simulink model "controlNN"  (R2020b)
settings: Solver=VariableStepAuto  StartTime=0.0  StopTime=50  RelTol=1e-3
undefined symbols (not defined in the file): DiscIntNeverNeededParam, FF_L, FF_R, initial_uspeed, Kih, Kir
libraries: neural x116, simulink x4, simulink_extras x3, dspsrcs4 x1, pid_lib x1
(part 2 of 5)

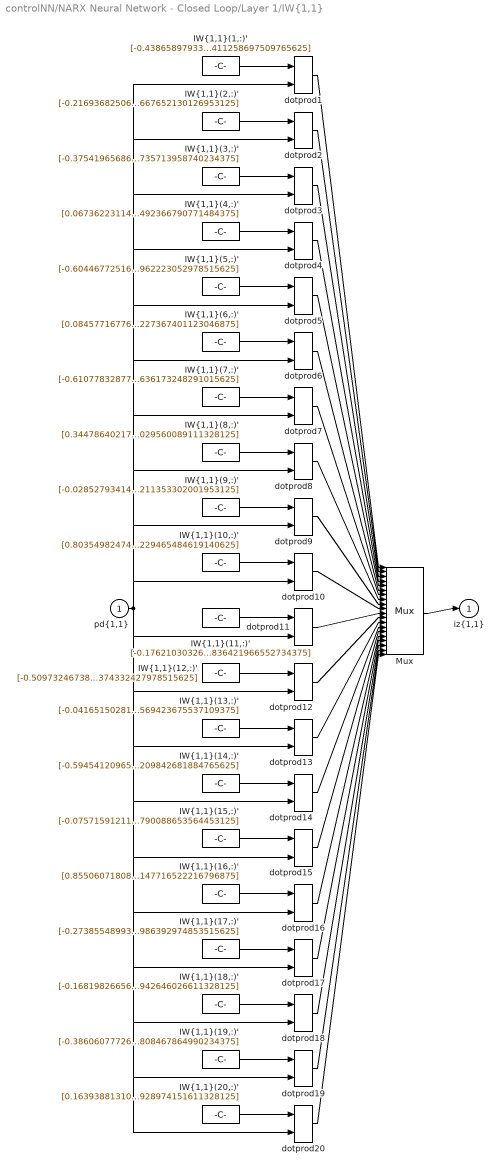
== system controlNN/NARX Neural Network - Closed Loop/Layer 1/IW{1,1} ==
  "pd{1,1}" : Inport  PortDimensions=4  SampleTime=0.1
      mask Display: e = 0.06;c1 = [120 230 180]/255;c2 = ([120 230 180]+0)/(256+128);c3 = ([120 230 180]+128)/(256+128);patch([0 1 1 0],[0 0 1 1],c1);patch([0 1 1 1-e 1-e 0+e],[0 0 1 1-e 0+e 0+e],c2);patch([0 0 1 1-e 0+e 0+e],[0 1 1 1-e 1-e 0+e],c3);plot([0 1 1 0 0],[0 0 1 1 0]);
  "IW{1,1}(1,:)'" : Constant  Value=[-0.4386589793372710488483789958991110324859619140625;-0.018740802820601483447138235760576208122074604034423828125;0.417644650165202413472087528134579770267009735107421875;-0.11303759033649586618341942312326864339411258697509765625]
      mask Display: e = 0.06;c1 = [120 150 230]/255;c2 = ([120 150 230]+0)/383;c3 = ([120 150 230]+128)/383;patch([0 1 1 0],[0 0 1 1],c1);patch([0 1 1 1-e 1-e 0+e],[0 0 1 1-e 0+e 0+e],c2);patch([0 0 1 1-e 0+e 0+e],[0 1 1 1-e 1-e 0+e],c3);plot([0 1 1 0 0],[0 0 1 1 0]);disp('Weights');
  "IW{1,1}(10,:)'" : Constant  Value=[0.8035498247491827950028664417914114892482757568359375;-0.852615893781887290714394112001173198223114013671875;0.029692839364198787832638259942541480995714664459228515625;0.131333870605793878727496348801651038229465484619140625]
      mask Display: e = 0.06;c1 = [120 150 230]/255;c2 = ([120 150 230]+0)/383;c3 = ([120 150 230]+128)/383;patch([0 1 1 0],[0 0 1 1],c1);patch([0 1 1 1-e 1-e 0+e],[0 0 1 1-e 0+e 0+e],c2);patch([0 0 1 1-e 0+e 0+e],[0 1 1 1-e 1-e 0+e],c3);plot([0 1 1 0 0],[0 0 1 1 0]);disp('Weights');
  "IW{1,1}(11,:)'" : Constant  Value=[-0.176210303269895229849595352789037860929965972900390625;0.3631567673090703163296666389214806258678436279296875;0.00443034452357003206979246812124983989633619785308837890625;-0.279013486365463359017979882992221973836421966552734375]
      mask Display: e = 0.06;c1 = [120 150 230]/255;c2 = ([120 150 230]+0)/383;c3 = ([120 150 230]+128)/383;patch([0 1 1 0],[0 0 1 1],c1);patch([0 1 1 1-e 1-e 0+e],[0 0 1 1-e 0+e 0+e],c2);patch([0 0 1 1-e 0+e 0+e],[0 1 1 1-e 1-e 0+e],c3);plot([0 1 1 0 0],[0 0 1 1 0]);disp('Weights');
  "IW{1,1}(12,:)'" : Constant  Value=[-0.50973246738134780908779930541641078889369964599609375;0.1274233060214269019905231061784434132277965545654296875;-0.03424515071449614478371614723073435015976428985595703125;-0.0299313497305035459972177847021157504059374332427978515625]
      mask Display: e = 0.06;c1 = [120 150 230]/255;c2 = ([120 150 230]+0)/383;c3 = ([120 150 230]+128)/383;patch([0 1 1 0],[0 0 1 1],c1);patch([0 1 1 1-e 1-e 0+e],[0 0 1 1-e 0+e 0+e],c2);patch([0 0 1 1-e 0+e 0+e],[0 1 1 1-e 1-e 0+e],c3);plot([0 1 1 0 0],[0 0 1 1 0]);disp('Weights');
  "IW{1,1}(13,:)'" : Constant  Value=[-0.041651502817647630128039537567019579000771045684814453125;-0.10168864752925420302798187321968725882470607757568359375;-0.14637329203365190277708052235539071261882781982421875;-0.3056214640627208378731438642716966569423675537109375]
      mask Display: e = 0.06;c1 = [120 150 230]/255;c2 = ([120 150 230]+0)/383;c3 = ([120 150 230]+128)/383;patch([0 1 1 0],[0 0 1 1],c1);patch([0 1 1 1-e 1-e 0+e],[0 0 1 1-e 0+e 0+e],c2);patch([0 0 1 1-e 0+e 0+e],[0 1 1 1-e 1-e 0+e],c3);plot([0 1 1 0 0],[0 0 1 1 0]);disp('Weights');
  "IW{1,1}(14,:)'" : Constant  Value=[-0.59454120965693724176759360489086247980594635009765625;0.187929342664180765165582442932645790278911590576171875;0.174064349978933885498832978555583395063877105712890625;-0.53969192686360278887747199405566789209842681884765625]
      mask Display: e = 0.06;c1 = [120 150 230]/255;c2 = ([120 150 230]+0)/383;c3 = ([120 150 230]+128)/383;patch([0 1 1 0],[0 0 1 1],c1);patch([0 1 1 1-e 1-e 0+e],[0 0 1 1-e 0+e 0+e],c2);patch([0 0 1 1-e 0+e 0+e],[0 1 1 1-e 1-e 0+e],c3);plot([0 1 1 0 0],[0 0 1 1 0]);disp('Weights');
  "IW{1,1}(15,:)'" : Constant  Value=[-0.07571591211695156975469700455505517311394214630126953125;0.407648907576858565704469583579339087009429931640625;0.017529421576475530397676294569464516825973987579345703125;-0.2305489952766562045116671697542187757790088653564453125]
      mask Display: e = 0.06;c1 = [120 150 230]/255;c2 = ([120 150 230]+0)/383;c3 = ([120 150 230]+128)/383;patch([0 1 1 0],[0 0 1 1],c1);patch([0 1 1 1-e 1-e 0+e],[0 0 1 1-e 0+e 0+e],c2);patch([0 0 1 1-e 0+e 0+e],[0 1 1 1-e 1-e 0+e],c3);plot([0 1 1 0 0],[0 0 1 1 0]);disp('Weights');
  "IW{1,1}(16,:)'" : Constant  Value=[0.8550607180854485900312056401162408292293548583984375;-0.76669221688588040652945210240432061254978179931640625;-0.330474331205291294022430292898206971585750579833984375;1.144481090073003581863986255484633147716522216796875]
      mask Display: e = 0.06;c1 = [120 150 230]/255;c2 = ([120 150 230]+0)/383;c3 = ([120 150 230]+128)/383;patch([0 1 1 0],[0 0 1 1],c1);patch([0 1 1 1-e 1-e 0+e],[0 0 1 1-e 0+e 0+e],c2);patch([0 0 1 1-e 0+e 0+e],[0 1 1 1-e 1-e 0+e],c3);plot([0 1 1 0 0],[0 0 1 1 0]);disp('Weights');
  "IW{1,1}(17,:)'" : Constant  Value=[-0.273855489939183183167870083707384765148162841796875;0.73849739533944214198157851569703780114650726318359375;-0.161805029543822309623379851473146118223667144775390625;-0.376344550552319800917899783598841167986392974853515625]
      mask Display: e = 0.06;c1 = [120 150 230]/255;c2 = ([120 150 230]+0)/383;c3 = ([120 150 230]+128)/383;patch([0 1 1 0],[0 0 1 1],c1);patch([0 1 1 1-e 1-e 0+e],[0 0 1 1-e 0+e 0+e],c2);patch([0 0 1 1-e 0+e 0+e],[0 1 1 1-e 1-e 0+e],c3);plot([0 1 1 0 0],[0 0 1 1 0]);disp('Weights');
  "IW{1,1}(18,:)'" : Constant  Value=[-0.1681982665624602024667666455570724792778491973876953125;0.1950333915332860268421200089505873620510101318359375;0.325788197182866390289035507521475665271282196044921875;0.38078155832405713443478134649922139942646026611328125]
      mask Display: e = 0.06;c1 = [120 150 230]/255;c2 = ([120 150 230]+0)/383;c3 = ([120 150 230]+128)/383;patch([0 1 1 0],[0 0 1 1],c1);patch([0 1 1 1-e 1-e 0+e],[0 0 1 1-e 0+e 0+e],c2);patch([0 0 1 1-e 0+e 0+e],[0 1 1 1-e 1-e 0+e],c3);plot([0 1 1 0 0],[0 0 1 1 0]);disp('Weights');
  "IW{1,1}(19,:)'" : Constant  Value=[-0.3860607772679796045878219956648536026477813720703125;0.005620361738486860138375167394997333758510649204254150390625;-0.2093565241992116632285814148417557589709758758544921875;0.203667618207004019748040946069522760808467864990234375]
      mask Display: e = 0.06;c1 = [120 150 230]/255;c2 = ([120 150 230]+0)/383;c3 = ([120 150 230]+128)/383;patch([0 1 1 0],[0 0 1 1],c1);patch([0 1 1 1-e 1-e 0+e],[0 0 1 1-e 0+e 0+e],c2);patch([0 0 1 1-e 0+e 0+e],[0 1 1 1-e 1-e 0+e],c3);plot([0 1 1 0 0],[0 0 1 1 0]);disp('Weights');
  "IW{1,1}(2,:)'" : Constant  Value=[-0.2169368250631043271159370533496257849037647247314453125;-0.10077498959220541896453227082020021043717861175537109375;0.2530416473236523078327309121959842741489410400390625;0.66912441916586662404853314001229591667652130126953125]
      mask Display: e = 0.06;c1 = [120 150 230]/255;c2 = ([120 150 230]+0)/383;c3 = ([120 150 230]+128)/383;patch([0 1 1 0],[0 0 1 1],c1);patch([0 1 1 1-e 1-e 0+e],[0 0 1 1-e 0+e 0+e],c2);patch([0 0 1 1-e 0+e 0+e],[0 1 1 1-e 1-e 0+e],c3);plot([0 1 1 0 0],[0 0 1 1 0]);disp('Weights');
  "IW{1,1}(20,:)'" : Constant  Value=[0.1639388131040236118440844848009874112904071807861328125;-0.11483736125112457837627033541139098815619945526123046875;-0.2099411749306478169874168315800488926470279693603515625;0.08683169221030291595742056642848183400928974151611328125]
      mask Display: e = 0.06;c1 = [120 150 230]/255;c2 = ([120 150 230]+0)/383;c3 = ([120 150 230]+128)/383;patch([0 1 1 0],[0 0 1 1],c1);patch([0 1 1 1-e 1-e 0+e],[0 0 1 1-e 0+e 0+e],c2);patch([0 0 1 1-e 0+e 0+e],[0 1 1 1-e 1-e 0+e],c3);plot([0 1 1 0 0],[0 0 1 1 0]);disp('Weights');
  "IW{1,1}(3,:)'" : Constant  Value=[-0.37541965686606160179650260033668018877506256103515625;-0.20153178909663049811484825113439001142978668212890625;-0.466435294275771183958312349204788915812969207763671875;0.33277599345324071489216066765948198735713958740234375]
      mask Display: e = 0.06;c1 = [120 150 230]/255;c2 = ([120 150 230]+0)/383;c3 = ([120 150 230]+128)/383;patch([0 1 1 0],[0 0 1 1],c1);patch([0 1 1 1-e 1-e 0+e],[0 0 1 1-e 0+e 0+e],c2);patch([0 0 1 1-e 0+e 0+e],[0 1 1 1-e 1-e 0+e],c3);plot([0 1 1 0 0],[0 0 1 1 0]);disp('Weights');
  "IW{1,1}(4,:)'" : Constant  Value=[0.0673622311467110268523583727073855698108673095703125;-0.486251970232177532782458229121402837336063385009765625;-0.06241567356591477822025382238280144520103931427001953125;0.402933162705098213418608565916656516492366790771484375]
      mask Display: e = 0.06;c1 = [120 150 230]/255;c2 = ([120 150 230]+0)/383;c3 = ([120 150 230]+128)/383;patch([0 1 1 0],[0 0 1 1],c1);patch([0 1 1 1-e 1-e 0+e],[0 0 1 1-e 0+e 0+e],c2);patch([0 0 1 1-e 0+e 0+e],[0 1 1 1-e 1-e 0+e],c3);plot([0 1 1 0 0],[0 0 1 1 0]);disp('Weights');
  "IW{1,1}(5,:)'" : Constant  Value=[-0.6044677251635601766821537239593453705310821533203125;0.59556534702274677162137095365324057638645172119140625;-0.2165999782456699274124645171468728221952915191650390625;-0.32745838498189228094048530692816711962223052978515625]
      mask Display: e = 0.06;c1 = [120 150 230]/255;c2 = ([120 150 230]+0)/383;c3 = ([120 150 230]+128)/383;patch([0 1 1 0],[0 0 1 1],c1);patch([0 1 1 1-e 1-e 0+e],[0 0 1 1-e 0+e 0+e],c2);patch([0 0 1 1-e 0+e 0+e],[0 1 1 1-e 1-e 0+e],c3);plot([0 1 1 0 0],[0 0 1 1 0]);disp('Weights');
  "IW{1,1}(6,:)'" : Constant  Value=[0.08457716776205737030380760188563726842403411865234375;0.164731897714957831180271341509069316089153289794921875;0.06115368927873300608499818054042407311499118804931640625;-0.162399602033176104765033187504741363227367401123046875]
      mask Display: e = 0.06;c1 = [120 150 230]/255;c2 = ([120 150 230]+0)/383;c3 = ([120 150 230]+128)/383;patch([0 1 1 0],[0 0 1 1],c1);patch([0 1 1 1-e 1-e 0+e],[0 0 1 1-e 0+e 0+e],c2);patch([0 0 1 1-e 0+e 0+e],[0 1 1 1-e 1-e 0+e],c3);plot([0 1 1 0 0],[0 0 1 1 0]);disp('Weights');
  "IW{1,1}(7,:)'" : Constant  Value=[-0.6107783287765347068898336146958172321319580078125;0.056990451234282736570069261006210581399500370025634765625;-0.164006181104764670042328589261160232126712799072265625;-0.0957481372975642897049652901841909624636173248291015625]
      mask Display: e = 0.06;c1 = [120 150 230]/255;c2 = ([120 150 230]+0)/383;c3 = ([120 150 230]+128)/383;patch([0 1 1 0],[0 0 1 1],c1);patch([0 1 1 1-e 1-e 0+e],[0 0 1 1-e 0+e 0+e],c2);patch([0 0 1 1-e 0+e 0+e],[0 1 1 1-e 1-e 0+e],c3);plot([0 1 1 0 0],[0 0 1 1 0]);disp('Weights');
  "IW{1,1}(8,:)'" : Constant  Value=[0.34478640217807143830697214070823974907398223876953125;-0.496796585967090920110678098353673703968524932861328125;-0.067509984111881971013957581817521713674068450927734375;0.3095067145511365414023430275847204029560089111328125]
      mask Display: e = 0.06;c1 = [120 150 230]/255;c2 = ([120 150 230]+0)/383;c3 = ([120 150 230]+128)/383;patch([0 1 1 0],[0 0 1 1],c1);patch([0 1 1 1-e 1-e 0+e],[0 0 1 1-e 0+e 0+e],c2);patch([0 0 1 1-e 0+e 0+e],[0 1 1 1-e 1-e 0+e],c3);plot([0 1 1 0 0],[0 0 1 1 0]);disp('Weights');
  "IW{1,1}(9,:)'" : Constant  Value=[-0.02852793414041586428364638550192466937005519866943359375;0.1993846370832842718190391906318836845457553863525390625;-0.1083183159449141730323873389352229423820972442626953125;-0.18780342166301100537140200685826130211353302001953125]
      mask Display: e = 0.06;c1 = [120 150 230]/255;c2 = ([120 150 230]+0)/383;c3 = ([120 150 230]+128)/383;patch([0 1 1 0],[0 0 1 1],c1);patch([0 1 1 1-e 1-e 0+e],[0 0 1 1-e 0+e 0+e],c2);patch([0 0 1 1-e 0+e 0+e],[0 1 1 1-e 1-e 0+e],c3);plot([0 1 1 0 0],[0 0 1 1 0]);disp('Weights');
  Mux : Mux  Inputs=20
      mask Display: e = 0.06;c1 = [120 150 230]/255;c2 = ([120 150 230]+0)/383;c3 = ([120 150 230]+128)/383;patch([0 1 1 0],[0 0 1 1],c1);patch([0 1 1 1-e 1-e 0+e],[0 0 1 1-e 0+e 0+e],c2);patch([0 0 1 1-e 0+e 0+e],[0 1 1 1-e 1-e 0+e],c3);plot([0 1 1 0 0],[0 0 1 1 0]);disp('Mux');
  dotprod{1..20} (20 alike) : neural/Weight Functions/dotprod
  "iz{1,1}" : Outport
      mask Display: e = 0.06;c1 = [120 230 180]/255;c2 = ([120 230 180]+0)/(256+128);c3 = ([120 230 180]+128)/(256+128);patch([0 1 1 0],[0 0 1 1],c1);patch([0 1 1 1-e 1-e 0+e],[0 0 1 1-e 0+e 0+e],c2);patch([0 0 1 1-e 0+e 0+e],[0 1 1 1-e 1-e 0+e],c3);plot([0 1 1 0 0],[0 0 1 1 0]);
  wires:
  "IW{1,1}(1,:)'"/1 -> dotprod1/1
  "pd{1,1}"/1 -> dotprod1/2, dotprod2/2, dotprod3/2, dotprod4/2, dotprod5/2, dotprod6/2, dotprod7/2, dotprod8/2, dotprod9/2, dotprod10/2, dotprod11/2, dotprod12/2, dotprod13/2, dotprod14/2, dotprod15/2, dotprod16/2, dotprod17/2, dotprod18/2, dotprod19/2, dotprod20/2
  dotprod1/1 -> Mux/1
  "IW{1,1}(2,:)'"/1 -> dotprod2/1
  dotprod2/1 -> Mux/2
  "IW{1,1}(3,:)'"/1 -> dotprod3/1
  dotprod3/1 -> Mux/3
  "IW{1,1}(4,:)'"/1 -> dotprod4/1
  dotprod4/1 -> Mux/4
  "IW{1,1}(5,:)'"/1 -> dotprod5/1
  dotprod5/1 -> Mux/5
  "IW{1,1}(6,:)'"/1 -> dotprod6/1
  dotprod6/1 -> Mux/6
  "IW{1,1}(7,:)'"/1 -> dotprod7/1
  dotprod7/1 -> Mux/7
  "IW{1,1}(8,:)'"/1 -> dotprod8/1
  dotprod8/1 -> Mux/8
  "IW{1,1}(9,:)'"/1 -> dotprod9/1
  dotprod9/1 -> Mux/9
  "IW{1,1}(10,:)'"/1 -> dotprod10/1
  dotprod10/1 -> Mux/10
  "IW{1,1}(11,:)'"/1 -> dotprod11/1
  dotprod11/1 -> Mux/11
  "IW{1,1}(12,:)'"/1 -> dotprod12/1
  dotprod12/1 -> Mux/12
  "IW{1,1}(13,:)'"/1 -> dotprod13/1
  dotprod13/1 -> Mux/13
  "IW{1,1}(14,:)'"/1 -> dotprod14/1
  dotprod14/1 -> Mux/14
  "IW{1,1}(15,:)'"/1 -> dotprod15/1
  dotprod15/1 -> Mux/15
  "IW{1,1}(16,:)'"/1 -> dotprod16/1
  dotprod16/1 -> Mux/16
  "IW{1,1}(17,:)'"/1 -> dotprod17/1
  dotprod17/1 -> Mux/17
  "IW{1,1}(18,:)'"/1 -> dotprod18/1
  dotprod18/1 -> Mux/18
  "IW{1,1}(19,:)'"/1 -> dotprod19/1
  dotprod19/1 -> Mux/19
  "IW{1,1}(20,:)'"/1 -> dotprod20/1
  dotprod20/1 -> Mux/20
  Mux/1 -> "iz{1,1}"/1

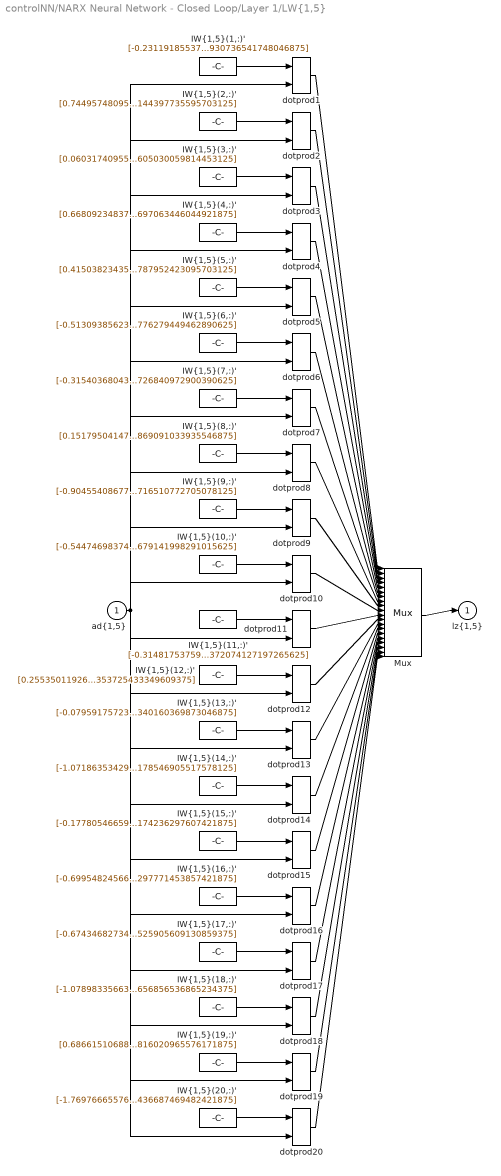
== system controlNN/NARX Neural Network - Closed Loop/Layer 1/LW{1,5} ==
  "ad{1,5}" : Inport  PortDimensions=9  SampleTime=0.1
      mask Display: e = 0.06;c1 = [120 230 180]/255;c2 = ([120 230 180]+0)/(256+128);c3 = ([120 230 180]+128)/(256+128);patch([0 1 1 0],[0 0 1 1],c1);patch([0 1 1 1-e 1-e 0+e],[0 0 1 1-e 0+e 0+e],c2);patch([0 0 1 1-e 0+e 0+e],[0 1 1 1-e 1-e 0+e],c3);plot([0 1 1 0 0],[0 0 1 1 0]);
  "IW{1,5}(1,:)'" : Constant  Value=[-0.2311918553757970062889626206015236675739288330078125;0.5221402736602007710331463385955430567264556884765625;0.0243916179590730301807166569005858036689460277557373046875;-0.217996142397916481403541411054902710020542144775390625;-0.1464474710870238005622212540401960723102092742919921875;0.5650549066626735505991518948576413094997406005859375;-0.023897965720476442574859987644231296144425868988037109375;0.11174950041300375780384257495825295336544513702392578125;0.73893306396338143127167086277040652930736541748046875]
      mask Display: e = 0.06;c1 = [120 150 230]/255;c2 = ([120 150 230]+0)/383;c3 = ([120 150 230]+128)/383;patch([0 1 1 0],[0 0 1 1],c1);patch([0 1 1 1-e 1-e 0+e],[0 0 1 1-e 0+e 0+e],c2);patch([0 0 1 1-e 0+e 0+e],[0 1 1 1-e 1-e 0+e],c3);plot([0 1 1 0 0],[0 0 1 1 0]);disp('weights');
  "IW{1,5}(10,:)'" : Constant  Value=[-0.544746983743852997150725059327669441699981689453125;-0.0208669004603495890359798892177423113025724887847900390625;-0.0390067613804046253722646042660926468670368194580078125;-0.284810235129842104218056419995264150202274322509765625;1.351958020913929914286200073547661304473876953125;0.162511610923024185648699813100392930209636688232421875;-0.22443140784391879538617331490968354046344757080078125;-0.06900460407357102143866001142669119872152805328369140625;0.8008568126875614812121284558088518679141998291015625]
      mask Display: e = 0.06;c1 = [120 150 230]/255;c2 = ([120 150 230]+0)/383;c3 = ([120 150 230]+128)/383;patch([0 1 1 0],[0 0 1 1],c1);patch([0 1 1 1-e 1-e 0+e],[0 0 1 1-e 0+e 0+e],c2);patch([0 0 1 1-e 0+e 0+e],[0 1 1 1-e 1-e 0+e],c3);plot([0 1 1 0 0],[0 0 1 1 0]);disp('weights');
  "IW{1,5}(11,:)'" : Constant  Value=[-0.3148175375952864119000196296838112175464630126953125;-0.0201252255988595106506178211702717817388474941253662109375;-0.041906260492351458946114206582933547906577587127685546875;0.3251339505202330837363433602149598300457000732421875;0.183494807709077945023778966060490347445011138916015625;-0.01587083282701005904069546659229672513902187347412109375;-0.270686784721715867352287432368029840290546417236328125;0.0331311256809694032465785085150855593383312225341796875;0.1110384185024998748847480101176188327372074127197265625]
      mask Display: e = 0.06;c1 = [120 150 230]/255;c2 = ([120 150 230]+0)/383;c3 = ([120 150 230]+128)/383;patch([0 1 1 0],[0 0 1 1],c1);patch([0 1 1 1-e 1-e 0+e],[0 0 1 1-e 0+e 0+e],c2);patch([0 0 1 1-e 0+e 0+e],[0 1 1 1-e 1-e 0+e],c3);plot([0 1 1 0 0],[0 0 1 1 0]);disp('weights');
  "IW{1,5}(12,:)'" : Constant  Value=[0.25535011926189488118410508832312189042568206787109375;-0.06781103850008314559705269175537978298962116241455078125;-0.1765333104449736401075909952851361595094203948974609375;-0.07995557032786904105847725077182985842227935791015625;-0.56790209529041202340948757409933023154735565185546875;0.12368783117214422750951285934206680394709110260009765625;-0.050807955374315115493200067930956720374524593353271484375;-0.1708000662816792358800199735924252308905124664306640625;-0.3310316189289499444470266098505817353725433349609375]
      mask Display: e = 0.06;c1 = [120 150 230]/255;c2 = ([120 150 230]+0)/383;c3 = ([120 150 230]+128)/383;patch([0 1 1 0],[0 0 1 1],c1);patch([0 1 1 1-e 1-e 0+e],[0 0 1 1-e 0+e 0+e],c2);patch([0 0 1 1-e 0+e 0+e],[0 1 1 1-e 1-e 0+e],c3);plot([0 1 1 0 0],[0 0 1 1 0]);disp('weights');
  "IW{1,5}(13,:)'" : Constant  Value=[-0.079591757232955473444491190093685872852802276611328125;0.26871266099311064134980142625863663852214813232421875;0.19483515376642579486343720418517477810382843017578125;0.2158877741672318439913880183667060919106006622314453125;-0.7479795700745845987711390989716164767742156982421875;0.64235516354538024774711857389775104820728302001953125;-0.301808244484936871732116969724302180111408233642578125;0.409133320230898822611464993315166793763637542724609375;-0.01345306195830124444678954631626766058616340160369873046875]
      mask Display: e = 0.06;c1 = [120 150 230]/255;c2 = ([120 150 230]+0)/383;c3 = ([120 150 230]+128)/383;patch([0 1 1 0],[0 0 1 1],c1);patch([0 1 1 1-e 1-e 0+e],[0 0 1 1-e 0+e 0+e],c2);patch([0 0 1 1-e 0+e 0+e],[0 1 1 1-e 1-e 0+e],c3);plot([0 1 1 0 0],[0 0 1 1 0]);disp('weights');
  "IW{1,5}(14,:)'" : Constant  Value=[-1.071863534293599595770274390815757215023040771484375;0.1989523045064365280865104068652726709842681884765625;0.220235805372647586164447375267627649009227752685546875;-0.41885820333493539724400989143759943544864654541015625;0.2410461404675325047808343015276477672159671783447265625;-0.0800863220582195278751669320627115666866302490234375;0.28295401326276181652730201676604337990283966064453125;0.72681780994764988435008490341715514659881591796875;-0.3208844679775921804321114905178546905517578125]
      mask Display: e = 0.06;c1 = [120 150 230]/255;c2 = ([120 150 230]+0)/383;c3 = ([120 150 230]+128)/383;patch([0 1 1 0],[0 0 1 1],c1);patch([0 1 1 1-e 1-e 0+e],[0 0 1 1-e 0+e 0+e],c2);patch([0 0 1 1-e 0+e 0+e],[0 1 1 1-e 1-e 0+e],c3);plot([0 1 1 0 0],[0 0 1 1 0]);disp('weights');
  "IW{1,5}(15,:)'" : Constant  Value=[-0.17780546659272411513796896542771719396114349365234375;-0.09782683516892017039356943541861255653202533721923828125;0.146761535994159475482234711307683028280735015869140625;0.08471415768842437132857270398744731210172176361083984375;0.54963220471845442016700644671800546348094940185546875;-0.0534051530097601478974667088550631888210773468017578125;0.07172658702519178752776696228465880267322063446044921875;-0.0810404904925203783960796499741263687610626220703125;-0.1615679641183165038409441649491782300174236297607421875]
      mask Display: e = 0.06;c1 = [120 150 230]/255;c2 = ([120 150 230]+0)/383;c3 = ([120 150 230]+128)/383;patch([0 1 1 0],[0 0 1 1],c1);patch([0 1 1 1-e 1-e 0+e],[0 0 1 1-e 0+e 0+e],c2);patch([0 0 1 1-e 0+e 0+e],[0 1 1 1-e 1-e 0+e],c3);plot([0 1 1 0 0],[0 0 1 1 0]);disp('weights');
  "IW{1,5}(16,:)'" : Constant  Value=[-0.6995482456630373047090643012779764831066131591796875;-0.52576189513835480671133382202242501080036163330078125;0.1860761240495697188546131428665830753743648529052734375;0.56796598824997868160124880887451581656932830810546875;0.91231789653880834833898916258476674556732177734375;0.171360138456032817799723488860763609409332275390625;-1.2741680689427834494154012645594775676727294921875;0.333742099312757556361930255661718547344207763671875;-0.0291920767385230144064234281131575698964297771453857421875]
      mask Display: e = 0.06;c1 = [120 150 230]/255;c2 = ([120 150 230]+0)/383;c3 = ([120 150 230]+128)/383;patch([0 1 1 0],[0 0 1 1],c1);patch([0 1 1 1-e 1-e 0+e],[0 0 1 1-e 0+e 0+e],c2);patch([0 0 1 1-e 0+e 0+e],[0 1 1 1-e 1-e 0+e],c3);plot([0 1 1 0 0],[0 0 1 1 0]);disp('weights');
  "IW{1,5}(17,:)'" : Constant  Value=[-0.67434682734431816708564610962639562785625457763671875;0.178838922670269628856232202451792545616626739501953125;-0.022826342936018338691805951157220988534390926361083984375;-0.2204262955518062894189057487892569042742252349853515625;0.785536261603020147248344073886983096599578857421875;-0.1615962577050045201332295619067735970020294189453125;-0.0093114199088808434490172061259727342985570430755615234375;-0.280812232310453990802301404983154498040676116943359375;-0.95914663710902414717196506899199448525905609130859375]
      mask Display: e = 0.06;c1 = [120 150 230]/255;c2 = ([120 150 230]+0)/383;c3 = ([120 150 230]+128)/383;patch([0 1 1 0],[0 0 1 1],c1);patch([0 1 1 1-e 1-e 0+e],[0 0 1 1-e 0+e 0+e],c2);patch([0 0 1 1-e 0+e 0+e],[0 1 1 1-e 1-e 0+e],c3);plot([0 1 1 0 0],[0 0 1 1 0]);disp('weights');
  "IW{1,5}(18,:)'" : Constant  Value=[-1.078983356633028467541635109228082001209259033203125;-0.152340207705443209107443180982954800128936767578125;-0.5027701143566332131484841738711111247539520263671875;0.060090279501787698113179914116699364967644214630126953125;-1.1640670189974822168466062066727317869663238525390625;-0.00749808428928296945292775177449584589339792728424072265625;0.12136923272946520402371106683858670294284820556640625;0.2732159578249688802742412008228711783885955810546875;-0.5690733337947315728655439670546911656856536865234375]
      mask Display: e = 0.06;c1 = [120 150 230]/255;c2 = ([120 150 230]+0)/383;c3 = ([120 150 230]+128)/383;patch([0 1 1 0],[0 0 1 1],c1);patch([0 1 1 1-e 1-e 0+e],[0 0 1 1-e 0+e 0+e],c2);patch([0 0 1 1-e 0+e 0+e],[0 1 1 1-e 1-e 0+e],c3);plot([0 1 1 0 0],[0 0 1 1 0]);disp('weights');
  "IW{1,5}(19,:)'" : Constant  Value=[0.6866151068830579351498499818262644112110137939453125;0.4167696411669290501578188923303969204425811767578125;-0.030303118363700608239863498738486669026315212249755859375;-0.109120263208447976222004172086599282920360565185546875;-0.250646056101163250406926863433909602463245391845703125;-0.0679626753089337676261294518553768284618854522705078125;0.09348235290963043120360254079059814102947711944580078125;0.061289170378221048685052352311686263419687747955322265625;-0.02061289046103102762241832124345819465816020965576171875]
      mask Display: e = 0.06;c1 = [120 150 230]/255;c2 = ([120 150 230]+0)/383;c3 = ([120 150 230]+128)/383;patch([0 1 1 0],[0 0 1 1],c1);patch([0 1 1 1-e 1-e 0+e],[0 0 1 1-e 0+e 0+e],c2);patch([0 0 1 1-e 0+e 0+e],[0 1 1 1-e 1-e 0+e],c3);plot([0 1 1 0 0],[0 0 1 1 0]);disp('weights');
  "IW{1,5}(2,:)'" : Constant  Value=[0.7449574809508783257427921853377483785152435302734375;-0.0807920145969898417792620648469892330467700958251953125;-0.399872941386871072477759980756673030555248260498046875;0.0155722487529322724253422194351514917798340320587158203125;0.25699801507336095252043151049292646348476409912109375;-0.81918424987524429692342664566240273416042327880859375;-0.0260157607196062103105393958912827656604349613189697265625;-0.08627645447615284179931904873228631913661956787109375;-0.16528831370213137308411432968568988144397735595703125]
      mask Display: e = 0.06;c1 = [120 150 230]/255;c2 = ([120 150 230]+0)/383;c3 = ([120 150 230]+128)/383;patch([0 1 1 0],[0 0 1 1],c1);patch([0 1 1 1-e 1-e 0+e],[0 0 1 1-e 0+e 0+e],c2);patch([0 0 1 1-e 0+e 0+e],[0 1 1 1-e 1-e 0+e],c3);plot([0 1 1 0 0],[0 0 1 1 0]);disp('weights');
  "IW{1,5}(20,:)'" : Constant  Value=[-1.769766655767905039198240046971477568149566650390625;0.265065305319353294866147052744054235517978668212890625;0.72061716294883415567795736933476291596889495849609375;0.105109097925626226999185064414632506668567657470703125;-1.2547638919973060911416951057617552578449249267578125;-0.930744205719426620504464153782464563846588134765625;-0.90781741721400066591485256140003912150859832763671875;-0.54251943368693933411606167283025570213794708251953125;0.956009447156883851448583300225436687469482421875]
      mask Display: e = 0.06;c1 = [120 150 230]/255;c2 = ([120 150 230]+0)/383;c3 = ([120 150 230]+128)/383;patch([0 1 1 0],[0 0 1 1],c1);patch([0 1 1 1-e 1-e 0+e],[0 0 1 1-e 0+e 0+e],c2);patch([0 0 1 1-e 0+e 0+e],[0 1 1 1-e 1-e 0+e],c3);plot([0 1 1 0 0],[0 0 1 1 0]);disp('weights');
  "IW{1,5}(3,:)'" : Constant  Value=[0.060317409551986424232072891982170403935015201568603515625;0.057931758825133954082797771434343303553760051727294921875;-0.224246217244899070930586049144039861857891082763671875;0.2025705673889336699833307875451282598078250885009765625;-0.457117882398095976004270823978004045784473419189453125;-0.49065460331151411477179635767242871224880218505859375;0.0829497760561776764642871739852125756442546844482421875;0.66372213128364088152721933511202223598957061767578125;0.181599632872566918440071503937360830605030059814453125]
      mask Display: e = 0.06;c1 = [120 150 230]/255;c2 = ([120 150 230]+0)/383;c3 = ([120 150 230]+128)/383;patch([0 1 1 0],[0 0 1 1],c1);patch([0 1 1 1-e 1-e 0+e],[0 0 1 1-e 0+e 0+e],c2);patch([0 0 1 1-e 0+e 0+e],[0 1 1 1-e 1-e 0+e],c3);plot([0 1 1 0 0],[0 0 1 1 0]);disp('weights');
  "IW{1,5}(4,:)'" : Constant  Value=[0.668092348372609112772124717594124376773834228515625;0.190434735620383654985943167048390023410320281982421875;-0.031049651140419111394752604837776743806898593902587890625;0.428427845714275778998825217058765701949596405029296875;-1.148271373911442072568434014101512730121612548828125;0.10706019914685087346395420127009856514632701873779296875;0.08499158049722900509781453592950128950178623199462890625;-0.1426987357925048327533801284516812302172183990478515625;0.08949018887541164424259676479778136126697063446044921875]
      mask Display: e = 0.06;c1 = [120 150 230]/255;c2 = ([120 150 230]+0)/383;c3 = ([120 150 230]+128)/383;patch([0 1 1 0],[0 0 1 1],c1);patch([0 1 1 1-e 1-e 0+e],[0 0 1 1-e 0+e 0+e],c2);patch([0 0 1 1-e 0+e 0+e],[0 1 1 1-e 1-e 0+e],c3);plot([0 1 1 0 0],[0 0 1 1 0]);disp('weights');
  "IW{1,5}(5,:)'" : Constant  Value=[0.41503823435174391764945767135941423475742340087890625;0.479217213303534617097056980128400027751922607421875;-0.187248295079222304426735945526161231100559234619140625;0.2297741142192083751982778494493686594069004058837890625;-0.2140682962172670567024823640167596749961376190185546875;0.0074521814198184356536902583911796682514250278472900390625;0.2446043967273450192578820860944688320159912109375;0.044939431962567118195028825766712543554604053497314453125;0.87727285150453948592286224084091372787952423095703125]
      mask Display: e = 0.06;c1 = [120 150 230]/255;c2 = ([120 150 230]+0)/383;c3 = ([120 150 230]+128)/383;patch([0 1 1 0],[0 0 1 1],c1);patch([0 1 1 1-e 1-e 0+e],[0 0 1 1-e 0+e 0+e],c2);patch([0 0 1 1-e 0+e 0+e],[0 1 1 1-e 1-e 0+e],c3);plot([0 1 1 0 0],[0 0 1 1 0]);disp('weights');
  "IW{1,5}(6,:)'" : Constant  Value=[-0.51309385623557723921095430341665633022785186767578125;-0.162822491033759064738006827610661275684833526611328125;-0.1862846771393187050858131215136381797492504119873046875;-0.1394360571084362343530216321596526540815830230712890625;0.86745887718931780074882453845930285751819610595703125;-0.0920634321942322142451331501433742232620716094970703125;0.2881839845735958416383937219507060945034027099609375;-0.03971301057516755939058583635414834134280681610107421875;-0.06850632423268400439386738298708223737776279449462890625]
      mask Display: e = 0.06;c1 = [120 150 230]/255;c2 = ([120 150 230]+0)/383;c3 = ([120 150 230]+128)/383;patch([0 1 1 0],[0 0 1 1],c1);patch([0 1 1 1-e 1-e 0+e],[0 0 1 1-e 0+e 0+e],c2);patch([0 0 1 1-e 0+e 0+e],[0 1 1 1-e 1-e 0+e],c3);plot([0 1 1 0 0],[0 0 1 1 0]);disp('weights');
  "IW{1,5}(7,:)'" : Constant  Value=[-0.315403680435300259876640893708099611103534698486328125;0.447418833107926350312055774338659830391407012939453125;0.1409179110875373452937964202646980993449687957763671875;0.0248654388815915637633846557719152770005166530609130859375;-0.278536351832139594808523952451650984585285186767578125;-0.0203761371768131811788027363263609004206955432891845703125;0.236005505788754288420960847361129708588123321533203125;0.60820436025920454614634991230559535324573516845703125;-0.266364352162722861638854965349310077726840972900390625]
      mask Display: e = 0.06;c1 = [120 150 230]/255;c2 = ([120 150 230]+0)/383;c3 = ([120 150 230]+128)/383;patch([0 1 1 0],[0 0 1 1],c1);patch([0 1 1 1-e 1-e 0+e],[0 0 1 1-e 0+e 0+e],c2);patch([0 0 1 1-e 0+e 0+e],[0 1 1 1-e 1-e 0+e],c3);plot([0 1 1 0 0],[0 0 1 1 0]);disp('weights');
  "IW{1,5}(8,:)'" : Constant  Value=[0.1517950414753181098692635941915796138346195220947265625;0.06229228492866152600004880923734162934124469757080078125;0.174757169160460856804917284534894861280918121337890625;0.29226110915448533233984562684781849384307861328125;-0.26617145796118013567621574111399240791797637939453125;0.0871827731143827444615368449376546777784824371337890625;-0.065957664919348124588083237540558911859989166259765625;0.53724447904414140975148939105565659701824188232421875;1.182587224416134841220582529786042869091033935546875]
      mask Display: e = 0.06;c1 = [120 150 230]/255;c2 = ([120 150 230]+0)/383;c3 = ([120 150 230]+128)/383;patch([0 1 1 0],[0 0 1 1],c1);patch([0 1 1 1-e 1-e 0+e],[0 0 1 1-e 0+e 0+e],c2);patch([0 0 1 1-e 0+e 0+e],[0 1 1 1-e 1-e 0+e],c3);plot([0 1 1 0 0],[0 0 1 1 0]);disp('weights');
  "IW{1,5}(9,:)'" : Constant  Value=[-0.90455408677829485242227747221477329730987548828125;0.20032806092079613602408016959088854491710662841796875;-0.0004573865565564604247252022961589545957394875586032867431640625;-0.388736708124420626830897163017652928829193115234375;0.553542832586063848765434158849529922008514404296875;-0.1341728246233460375425039501351420767605304718017578125;0.041863798129217498489307303088935441337525844573974609375;-0.403254305658925449318275013865786604583263397216796875;0.1239893703528594237628368546211277134716510772705078125]
      mask Display: e = 0.06;c1 = [120 150 230]/255;c2 = ([120 150 230]+0)/383;c3 = ([120 150 230]+128)/383;patch([0 1 1 0],[0 0 1 1],c1);patch([0 1 1 1-e 1-e 0+e],[0 0 1 1-e 0+e 0+e],c2);patch([0 0 1 1-e 0+e 0+e],[0 1 1 1-e 1-e 0+e],c3);plot([0 1 1 0 0],[0 0 1 1 0]);disp('weights');
  Mux : Mux  Inputs=20
      mask Display: e = 0.06;c1 = [120 150 230]/255;c2 = ([120 150 230]+0)/383;c3 = ([120 150 230]+128)/383;patch([0 1 1 0],[0 0 1 1],c1);patch([0 1 1 1-e 1-e 0+e],[0 0 1 1-e 0+e 0+e],c2);patch([0 0 1 1-e 0+e 0+e],[0 1 1 1-e 1-e 0+e],c3);plot([0 1 1 0 0],[0 0 1 1 0]);disp('Mux');
  dotprod{1..20} (20 alike) : neural/Weight Functions/dotprod
  "lz{1,5}" : Outport
      mask Display: e = 0.06;c1 = [120 230 180]/255;c2 = ([120 230 180]+0)/(256+128);c3 = ([120 230 180]+128)/(256+128);patch([0 1 1 0],[0 0 1 1],c1);patch([0 1 1 1-e 1-e 0+e],[0 0 1 1-e 0+e 0+e],c2);patch([0 0 1 1-e 0+e 0+e],[0 1 1 1-e 1-e 0+e],c3);plot([0 1 1 0 0],[0 0 1 1 0]);
  wires:
  "IW{1,5}(1,:)'"/1 -> dotprod1/1
  "ad{1,5}"/1 -> dotprod1/2, dotprod2/2, dotprod3/2, dotprod4/2, dotprod5/2, dotprod6/2, dotprod7/2, dotprod8/2, dotprod9/2, dotprod10/2, dotprod11/2, dotprod12/2, dotprod13/2, dotprod14/2, dotprod15/2, dotprod16/2, dotprod17/2, dotprod18/2, dotprod19/2, dotprod20/2
  dotprod1/1 -> Mux/1
  "IW{1,5}(2,:)'"/1 -> dotprod2/1
  dotprod2/1 -> Mux/2
  "IW{1,5}(3,:)'"/1 -> dotprod3/1
  dotprod3/1 -> Mux/3
  "IW{1,5}(4,:)'"/1 -> dotprod4/1
  dotprod4/1 -> Mux/4
  "IW{1,5}(5,:)'"/1 -> dotprod5/1
  dotprod5/1 -> Mux/5
  "IW{1,5}(6,:)'"/1 -> dotprod6/1
  dotprod6/1 -> Mux/6
  "IW{1,5}(7,:)'"/1 -> dotprod7/1
  dotprod7/1 -> Mux/7
  "IW{1,5}(8,:)'"/1 -> dotprod8/1
  dotprod8/1 -> Mux/8
  "IW{1,5}(9,:)'"/1 -> dotprod9/1
  dotprod9/1 -> Mux/9
  "IW{1,5}(10,:)'"/1 -> dotprod10/1
  dotprod10/1 -> Mux/10
  "IW{1,5}(11,:)'"/1 -> dotprod11/1
  dotprod11/1 -> Mux/11
  "IW{1,5}(12,:)'"/1 -> dotprod12/1
  dotprod12/1 -> Mux/12
  "IW{1,5}(13,:)'"/1 -> dotprod13/1
  dotprod13/1 -> Mux/13
  "IW{1,5}(14,:)'"/1 -> dotprod14/1
  dotprod14/1 -> Mux/14
  "IW{1,5}(15,:)'"/1 -> dotprod15/1
  dotprod15/1 -> Mux/15
  "IW{1,5}(16,:)'"/1 -> dotprod16/1
  dotprod16/1 -> Mux/16
  "IW{1,5}(17,:)'"/1 -> dotprod17/1
  dotprod17/1 -> Mux/17
  "IW{1,5}(18,:)'"/1 -> dotprod18/1
  dotprod18/1 -> Mux/18
  "IW{1,5}(19,:)'"/1 -> dotprod19/1
  dotprod19/1 -> Mux/19
  "IW{1,5}(20,:)'"/1 -> dotprod20/1
  dotprod20/1 -> Mux/20
  Mux/1 -> "lz{1,5}"/1

== system controlNN/NARX Neural Network - Closed Loop/Layer 2/Delays 1 ==
  "p{2}" : Inport  PortDimensions=20  SampleTime=0.1
      mask Display: e = 0.06;c1 = [120 230 180]/255;c2 = ([120 230 180]+0)/(256+128);c3 = ([120 230 180]+128)/(256+128);patch([0 1 1 0],[0 0 1 1],c1);patch([0 1 1 1-e 1-e 0+e],[0 0 1 1-e 0+e 0+e],c2);patch([0 0 1 1-e 0+e 0+e],[0 1 1 1-e 1-e 0+e],c3);plot([0 1 1 0 0],[0 0 1 1 0]);
  mux : Mux  Inputs=1
      mask Display: e = 0.06;c1 = [120 150 230]/255;c2 = ([120 150 230]+0)/383;c3 = ([120 150 230]+128)/383;patch([0 1 1 0],[0 0 1 1],c1);patch([0 1 1 1-e 1-e 0+e],[0 0 1 1-e 0+e 0+e],c2);patch([0 0 1 1-e 0+e 0+e],[0 1 1 1-e 1-e 0+e],c3);plot([0 1 1 0 0],[0 0 1 1 0]);disp('Mux')
  "pd{2,1}" : Outport
      mask Display: e = 0.06;c1 = [120 230 180]/255;c2 = ([120 230 180]+0)/(256+128);c3 = ([120 230 180]+128)/(256+128);patch([0 1 1 0],[0 0 1 1],c1);patch([0 1 1 1-e 1-e 0+e],[0 0 1 1-e 0+e 0+e],c2);patch([0 0 1 1-e 0+e 0+e],[0 1 1 1-e 1-e 0+e],c3);plot([0 1 1 0 0],[0 0 1 1 0]);
  wires:
  "p{2}"/1 -> mux/1
  mux/1 -> "pd{2,1}"/1
